simulink model "stdp_pattern3x3_training_2023noclock"  (R2024a)
settings: Solver=FixedStepAuto  StartTime=0.0  StopTime=2  FixedStep=0.000005  RelTol=1e-3
model workspace (MAT data in the model file):
  part1_v1 = 1
values from neighbouring files (symbols this model uses):
  full_pattern = load('Pattern4_250.CSV')    [model_setup4.m]
  max_weight2 = 255    [model_setup4.m]
  min_weight2 = 150    [model_setup4.m]
  Th_control_time2 = 0.02    [model_setup4.m]    (also in model_setup_test.m = 2)
  Th_minus_count2 = 10    [model_setup4.m]    (also in model_setup_test.m = 5)
  Th_plus_count2 = 20    [model_setup4.m]    (also in model_setup_test.m)
libraries: simulink x1
(part 9 of 9)

== matlab function stdp_pattern3x3_training_2023noclock/Post_Neuron1/MATLAB Function7 ==
  data: rc input; lateral_inhibition input; t input; inhibition_potential output
function inhibition_potential = fcn(rc, lateral_inhibition, t)

inhibition_potential = -lateral_inhibition * (exp(-(t)*rc));

== matlab function stdp_pattern3x3_training_2023noclock/Neuron1/MATLAB Function4 ==
  data: membrane_state input; t input; membrane_potential output
function membrane_potential = fcn(membrane_state, t)

membrane_potential = (membrane_state) * (exp(-(t)*0.015));

== matlab function stdp_pattern3x3_training_2023noclock/Neuron1/MATLAB Function5 ==
  data: t input; membrane_state input; membrane_potential output
function membrane_potential = fcn(t, membrane_state)

membrane_potential = (membrane_state) * 2.361128*(exp(-(t)*0.09)-0.6*exp(-(t+1)*0.04)) ;

== matlab function stdp_pattern3x3_training_2023noclock/Neuron1/Subsystem3/MATLAB Function ==
  data: u input; y output; min input; max input
function y = fcn(u, min, max)

if u<=min
    y=min;
elseif u>=max
    y=max;
else
    y=u;
end

== matlab function stdp_pattern3x3_training_2023noclock/Neuron5/MATLAB Function3 ==
  data: u input; y output
function y = fcn(u)

if u>=0
    y=1;
else
    y=0;
end

== matlab function stdp_pattern3x3_training_2023noclock/Neuron1/Subsystem3/MATLAB Function2 ==
  data: init_th input; y output; neuron_num input; before_threshold input
function y = fcn(init_th, neuron_num, before_threshold)

persistent n;

if isempty(n)
    n=init_th(neuron_num);
else
    n=before_threshold;
end

y=n;

== matlab function stdp_pattern3x3_training_2023noclock/Synapse1/rc_add2 ==
  data: tx input; initial_LTP input; pre_trace output; tau_LTP input
% rc_add2 (pre trace) - RC를 tau로 해석
function pre_trace = fcn(tx, initial_LTP, tau_LTP)
A   = initial_LTP(end);
tau = max(tau_LTP(end), eps);
pre_trace = A * exp(-tx / tau);

== matlab function stdp_pattern3x3_training_2023noclock/Subsystem1/MATLAB Function ==
  data: data input; y output; i input
function y = fcn(data, i)

j=1+i;
 y=data(j,:);
          

   
end

== matlab function stdp_pattern3x3_training_2023noclock/Neuron5/MATLAB Function4 ==
  data: membrane_state input; t input; membrane_potential output
function membrane_potential = fcn(membrane_state, t)

membrane_potential = (membrane_state) * (exp(-(t)*0.015));

== matlab function stdp_pattern3x3_training_2023noclock/Neuron5/MATLAB Function5 ==
  data: t input; membrane_state input; membrane_potential output
function membrane_potential = fcn(t, membrane_state)

membrane_potential = (membrane_state) * 2.361128*(exp(-(t)*0.09)-0.6*exp(-(t+1)*0.04)) ;

== matlab function stdp_pattern3x3_training_2023noclock/Neuron5/Subsystem3/MATLAB Function ==
  data: u input; y output; min input; max input
function y = fcn(u, min, max)

if u<=min
    y=min;
elseif u>=max
    y=max;
else
    y=u;
end

== matlab function stdp_pattern3x3_training_2023noclock/Neuron5/Subsystem3/MATLAB Function2 ==
  data: init_th input; y output; neuron_num input; before_threshold input
function y = fcn(init_th, neuron_num, before_threshold)

persistent n;

if isempty(n)
    n=init_th(neuron_num);
else
    n=before_threshold;
end

y=n;

== matlab function stdp_pattern3x3_training_2023noclock/Neuron6/MATLAB Function3 ==
  data: u input; y output
function y = fcn(u)

if u>=0
    y=1;
else
    y=0;
end

== matlab function stdp_pattern3x3_training_2023noclock/Neuron2/MATLAB Function3 ==
  data: u input; y output
function y = fcn(u)

if u>=0
    y=1;
else
    y=0;
end

== matlab function stdp_pattern3x3_training_2023noclock/Neuron6/MATLAB Function4 ==
  data: membrane_state input; t input; membrane_potential output
function membrane_potential = fcn(membrane_state, t)

membrane_potential = (membrane_state) * (exp(-(t)*0.015));

== matlab function stdp_pattern3x3_training_2023noclock/Neuron6/MATLAB Function5 ==
  data: t input; membrane_state input; membrane_potential output
function membrane_potential = fcn(t, membrane_state)

membrane_potential = (membrane_state) * 2.361128*(exp(-(t)*0.09)-0.6*exp(-(t+1)*0.04)) ;

== matlab function stdp_pattern3x3_training_2023noclock/Post_Neuron2/MATLAB Function3 ==
  data: membrane_state input; t input; membrane_potential output
function membrane_potential = fcn(membrane_state, t)

membrane_potential = (membrane_state) * (exp(-(t)*0.015));

== matlab function stdp_pattern3x3_training_2023noclock/Post_Neuron2/MATLAB Function4 ==
  data: t input; membrane_state input; membrane_potential output
function membrane_potential = fcn(t, membrane_state)

membrane_potential = (membrane_state) * 2.361128*(exp(-(t)*0.09)-0.6*exp(-(t+1)*0.04)) ;

== matlab function stdp_pattern3x3_training_2023noclock/Post_Neuron2/MATLAB Function7 ==
  data: rc input; lateral_inhibition input; t input; inhibition_potential output
function inhibition_potential = fcn(rc, lateral_inhibition, t)

inhibition_potential = -lateral_inhibition * (exp(-(t)*rc));

== matlab function stdp_pattern3x3_training_2023noclock/Post_Neuron2/Subsystem3/MATLAB Function ==
  data: u input; y output; min input; max input
function y = fcn(u, min, max)

if u<=min
    y=min;
elseif u>=max
    y=max;
else
    y=u;
end

== matlab function stdp_pattern3x3_training_2023noclock/Post_Neuron2/Subsystem3/MATLAB Function2 ==
  data: init_th input; y output; neuron_num input; before_threshold input
function y = fcn(init_th, neuron_num, before_threshold)

persistent n;

if isempty(n)
    n=init_th(neuron_num);
else
    n=before_threshold;
end

y=n;

== matlab function stdp_pattern3x3_training_2023noclock/Post_Neuron3/MATLAB Function1 ==
  data: u input; y output
function y = fcn(u)

if u>=0
    y=1;
else
    y=0;
end

== matlab function stdp_pattern3x3_training_2023noclock/Neuron2/MATLAB Function4 ==
  data: membrane_state input; t input; membrane_potential output
function membrane_potential = fcn(membrane_state, t)

membrane_potential = (membrane_state) * (exp(-(t)*0.015));

== matlab function stdp_pattern3x3_training_2023noclock/Post_Neuron3/MATLAB Function2 ==
  data: u input; y output
function y = fcn(u)
persistent k;
if isempty(k)
    k=0;
elseif u>0
    k=1;
end

y=k;

== matlab function stdp_pattern3x3_training_2023noclock/Post_Neuron3/MATLAB Function3 ==
  data: membrane_state input; t input; membrane_potential output
function membrane_potential = fcn(membrane_state, t)

membrane_potential = (membrane_state) * (exp(-(t)*0.015));

== matlab function stdp_pattern3x3_training_2023noclock/Post_Neuron3/MATLAB Function4 ==
  data: t input; membrane_state input; membrane_potential output
function membrane_potential = fcn(t, membrane_state)

membrane_potential = (membrane_state) * 2.361128*(exp(-(t)*0.09)-0.6*exp(-(t+1)*0.04)) ;

== matlab function stdp_pattern3x3_training_2023noclock/Post_Neuron3/MATLAB Function7 ==
  data: rc input; lateral_inhibition input; t input; inhibition_potential output
function inhibition_potential = fcn(rc, lateral_inhibition, t)

inhibition_potential = -lateral_inhibition * (exp(-(t)*rc));

== matlab function stdp_pattern3x3_training_2023noclock/Neuron6/Subsystem3/MATLAB Function ==
  data: u input; y output; min input; max input
function y = fcn(u, min, max)

if u<=min
    y=min;
elseif u>=max
    y=max;
else
    y=u;
end

== matlab function stdp_pattern3x3_training_2023noclock/Neuron6/Subsystem3/MATLAB Function2 ==
  data: init_th input; y output; neuron_num input; before_threshold input
function y = fcn(init_th, neuron_num, before_threshold)

persistent n;

if isempty(n)
    n=init_th(neuron_num);
else
    n=before_threshold;
end

y=n;

== matlab function stdp_pattern3x3_training_2023noclock/Synapse2/MATLAB Function1 ==
  data: init_weight input; y output; synapse_num input; before_weight input
function y = fcn(init_weight, synapse_num, before_weight)

persistent n;

if isempty(n)
    n=init_weight(synapse_num);
elseif before_weight>0
    n=before_weight;
end

y=n;

== matlab function stdp_pattern3x3_training_2023noclock/Synapse2/rc_add1 ==
  data: ty input; initial_LTD input; post_trace output; tau_LTD input
% rc_add1 (post trace) - RC를 tau로 해석
function post_trace = fcn(ty, initial_LTD, tau_LTD)
A   = initial_LTD(end);
tau = max(tau_LTD(end), eps);
post_trace = -A * exp(-ty / tau);

== matlab function stdp_pattern3x3_training_2023noclock/Synapse2/rc_add2 ==
  data: tx input; initial_LTP input; pre_trace output; tau_LTP input
% rc_add2 (pre trace) - RC를 tau로 해석
function pre_trace = fcn(tx, initial_LTP, tau_LTP)
A   = initial_LTP(end);
tau = max(tau_LTP(end), eps);
pre_trace = A * exp(-tx / tau);

== matlab function stdp_pattern3x3_training_2023noclock/Synapse3/MATLAB Function1 ==
  data: init_weight input; y output; synapse_num input; before_weight input
function y = fcn(init_weight, synapse_num, before_weight)

persistent n;

if isempty(n)
    n=init_weight(synapse_num);
elseif before_weight>0
    n=before_weight;
end

y=n;

== matlab function stdp_pattern3x3_training_2023noclock/Neuron2/MATLAB Function5 ==
  data: t input; membrane_state input; membrane_potential output
function membrane_potential = fcn(t, membrane_state)

membrane_potential = (membrane_state) * 2.361128*(exp(-(t)*0.09)-0.6*exp(-(t+1)*0.04)) ;

== matlab function stdp_pattern3x3_training_2023noclock/Synapse3/rc_add1 ==
  data: ty input; initial_LTD input; post_trace output; tau_LTD input
% rc_add1 (post trace) - RC를 tau로 해석
function post_trace = fcn(ty, initial_LTD, tau_LTD)
A   = initial_LTD(end);
tau = max(tau_LTD(end), eps);
post_trace = -A * exp(-ty / tau);

== matlab function stdp_pattern3x3_training_2023noclock/Synapse3/rc_add2 ==
  data: tx input; initial_LTP input; pre_trace output; tau_LTP input
% rc_add2 (pre trace) - RC를 tau로 해석
function pre_trace = fcn(tx, initial_LTP, tau_LTP)
A   = initial_LTP(end);
tau = max(tau_LTP(end), eps);
pre_trace = A * exp(-tx / tau);

== matlab function stdp_pattern3x3_training_2023noclock/Synapse4/MATLAB Function1 ==
  data: init_weight input; y output; synapse_num input; before_weight input
function y = fcn(init_weight, synapse_num, before_weight)

persistent n;

if isempty(n)
    n=init_weight(synapse_num);
elseif before_weight>0
    n=before_weight;
end

y=n;

== matlab function stdp_pattern3x3_training_2023noclock/Synapse4/rc_add1 ==
  data: ty input; initial_LTD input; post_trace output; tau_LTD input
% rc_add1 (post trace) - RC를 tau로 해석
function post_trace = fcn(ty, initial_LTD, tau_LTD)
A   = initial_LTD(end);
tau = max(tau_LTD(end), eps);
post_trace = -A * exp(-ty / tau);

== matlab function stdp_pattern3x3_training_2023noclock/Synapse4/rc_add2 ==
  data: tx input; initial_LTP input; pre_trace output; tau_LTP input
% rc_add2 (pre trace) - RC를 tau로 해석
function pre_trace = fcn(tx, initial_LTP, tau_LTP)
A   = initial_LTP(end);
tau = max(tau_LTP(end), eps);
pre_trace = A * exp(-tx / tau);

== matlab function stdp_pattern3x3_training_2023noclock/Synapse5/MATLAB Function1 ==
  data: init_weight input; y output; synapse_num input; before_weight input
function y = fcn(init_weight, synapse_num, before_weight)

persistent n;

if isempty(n)
    n=init_weight(synapse_num);
elseif before_weight>0
    n=before_weight;
end

y=n;

== matlab function stdp_pattern3x3_training_2023noclock/Synapse5/rc_add1 ==
  data: ty input; initial_LTD input; post_trace output; tau_LTD input
% rc_add1 (post trace) - RC를 tau로 해석
function post_trace = fcn(ty, initial_LTD, tau_LTD)
A   = initial_LTD(end);
tau = max(tau_LTD(end), eps);
post_trace = -A * exp(-ty / tau);

== matlab function stdp_pattern3x3_training_2023noclock/Synapse5/rc_add2 ==
  data: tx input; initial_LTP input; pre_trace output; tau_LTP input
% rc_add2 (pre trace) - RC를 tau로 해석
function pre_trace = fcn(tx, initial_LTP, tau_LTP)
A   = initial_LTP(end);
tau = max(tau_LTP(end), eps);
pre_trace = A * exp(-tx / tau);

== matlab function stdp_pattern3x3_training_2023noclock/Synapse6/MATLAB Function1 ==
  data: init_weight input; y output; synapse_num input; before_weight input
function y = fcn(init_weight, synapse_num, before_weight)

persistent n;

if isempty(n)
    n=init_weight(synapse_num);
elseif before_weight>0
    n=before_weight;
end

y=n;

== matlab function stdp_pattern3x3_training_2023noclock/Post_Neuron2/MATLAB Function1 ==
  data: u input; y output
function y = fcn(u)

if u>=0
    y=1;
else
    y=0;
end

== matlab function stdp_pattern3x3_training_2023noclock/Synapse6/rc_add1 ==
  data: ty input; initial_LTD input; post_trace output; tau_LTD input
% rc_add1 (post trace) - RC를 tau로 해석
function post_trace = fcn(ty, initial_LTD, tau_LTD)
A   = initial_LTD(end);
tau = max(tau_LTD(end), eps);
post_trace = -A * exp(-ty / tau);

== matlab function stdp_pattern3x3_training_2023noclock/Synapse6/rc_add2 ==
  data: tx input; initial_LTP input; pre_trace output; tau_LTP input
% rc_add2 (pre trace) - RC를 tau로 해석
function pre_trace = fcn(tx, initial_LTP, tau_LTP)
A   = initial_LTP(end);
tau = max(tau_LTP(end), eps);
pre_trace = A * exp(-tx / tau);

== matlab function stdp_pattern3x3_training_2023noclock/Synapse7/MATLAB Function1 ==
  data: init_weight input; y output; synapse_num input; before_weight input
function y = fcn(init_weight, synapse_num, before_weight)

persistent n;

if isempty(n)
    n=init_weight(synapse_num);
elseif before_weight>0
    n=before_weight;
end

y=n;

== matlab function stdp_pattern3x3_training_2023noclock/Synapse7/rc_add1 ==
  data: ty input; initial_LTD input; post_trace output; tau_LTD input
% rc_add1 (post trace) - RC를 tau로 해석
function post_trace = fcn(ty, initial_LTD, tau_LTD)
A   = initial_LTD(end);
tau = max(tau_LTD(end), eps);
post_trace = -A * exp(-ty / tau);

== matlab function stdp_pattern3x3_training_2023noclock/Synapse7/rc_add2 ==
  data: tx input; initial_LTP input; pre_trace output; tau_LTP input
% rc_add2 (pre trace) - RC를 tau로 해석
function pre_trace = fcn(tx, initial_LTP, tau_LTP)
A   = initial_LTP(end);
tau = max(tau_LTP(end), eps);
pre_trace = A * exp(-tx / tau);

== matlab function stdp_pattern3x3_training_2023noclock/Synapse8/MATLAB Function1 ==
  data: init_weight input; y output; synapse_num input; before_weight input
function y = fcn(init_weight, synapse_num, before_weight)

persistent n;

if isempty(n)
    n=init_weight(synapse_num);
elseif before_weight>0
    n=before_weight;
end

y=n;

== matlab function stdp_pattern3x3_training_2023noclock/Synapse8/rc_add1 ==
  data: ty input; initial_LTD input; post_trace output; tau_LTD input
% rc_add1 (post trace) - RC를 tau로 해석
function post_trace = fcn(ty, initial_LTD, tau_LTD)
A   = initial_LTD(end);
tau = max(tau_LTD(end), eps);
post_trace = -A * exp(-ty / tau);

== matlab function stdp_pattern3x3_training_2023noclock/Post_Neuron2/MATLAB Function2 ==
  data: u input; y output
function y = fcn(u)
persistent k;
if isempty(k)
    k=0;
elseif u>0
    k=1;
end

y=k;

== matlab function stdp_pattern3x3_training_2023noclock/Synapse8/rc_add2 ==
  data: tx input; initial_LTP input; pre_trace output; tau_LTP input
% rc_add2 (pre trace) - RC를 tau로 해석
function pre_trace = fcn(tx, initial_LTP, tau_LTP)
A   = initial_LTP(end);
tau = max(tau_LTP(end), eps);
pre_trace = A * exp(-tx / tau);

== matlab function stdp_pattern3x3_training_2023noclock/Synapse9/MATLAB Function1 ==
  data: init_weight input; y output; synapse_num input; before_weight input
function y = fcn(init_weight, synapse_num, before_weight)

persistent n;

if isempty(n)
    n=init_weight(synapse_num);
elseif before_weight>0
    n=before_weight;
end

y=n;

== matlab function stdp_pattern3x3_training_2023noclock/Synapse9/rc_add1 ==
  data: ty input; initial_LTD input; post_trace output; tau_LTD input
% rc_add1 (post trace) - RC를 tau로 해석
function post_trace = fcn(ty, initial_LTD, tau_LTD)
A   = initial_LTD(end);
tau = max(tau_LTD(end), eps);
post_trace = -A * exp(-ty / tau);

== matlab function stdp_pattern3x3_training_2023noclock/Synapse9/rc_add2 ==
  data: tx input; initial_LTP input; pre_trace output; tau_LTP input
% rc_add2 (pre trace) - RC를 tau로 해석
function pre_trace = fcn(tx, initial_LTP, tau_LTP)
A   = initial_LTP(end);
tau = max(tau_LTP(end), eps);
pre_trace = A * exp(-tx / tau);

== matlab function stdp_pattern3x3_training_2023noclock/Synapse10/MATLAB Function1 ==
  data: init_weight input; y output; synapse_num input; before_weight input
function y = fcn(init_weight, synapse_num, before_weight)

persistent n;

if isempty(n)
    n=init_weight(synapse_num);
elseif before_weight>0
    n=before_weight;
end

y=n;

== matlab function stdp_pattern3x3_training_2023noclock/Synapse10/rc_add1 ==
  data: ty input; initial_LTD input; post_trace output; tau_LTD input
% rc_add1 (post trace) - RC를 tau로 해석
function post_trace = fcn(ty, initial_LTD, tau_LTD)
A   = initial_LTD(end);
tau = max(tau_LTD(end), eps);
post_trace = -A * exp(-ty / tau);

== matlab function stdp_pattern3x3_training_2023noclock/Synapse10/rc_add2 ==
  data: tx input; initial_LTP input; pre_trace output; tau_LTP input
% rc_add2 (pre trace) - RC를 tau로 해석
function pre_trace = fcn(tx, initial_LTP, tau_LTP)
A   = initial_LTP(end);
tau = max(tau_LTP(end), eps);
pre_trace = A * exp(-tx / tau);

== matlab function stdp_pattern3x3_training_2023noclock/Synapse11/MATLAB Function1 ==
  data: init_weight input; y output; synapse_num input; before_weight input
function y = fcn(init_weight, synapse_num, before_weight)

persistent n;

if isempty(n)
    n=init_weight(synapse_num);
elseif before_weight>0
    n=before_weight;
end

y=n;

== matlab function stdp_pattern3x3_training_2023noclock/Neuron2/Subsystem3/MATLAB Function ==
  data: u input; y output; min input; max input
function y = fcn(u, min, max)

if u<=min
    y=min;
elseif u>=max
    y=max;
else
    y=u;
end

== matlab function stdp_pattern3x3_training_2023noclock/Synapse11/rc_add1 ==
  data: ty input; initial_LTD input; post_trace output; tau_LTD input
% rc_add1 (post trace) - RC를 tau로 해석
function post_trace = fcn(ty, initial_LTD, tau_LTD)
A   = initial_LTD(end);
tau = max(tau_LTD(end), eps);
post_trace = -A * exp(-ty / tau);

== matlab function stdp_pattern3x3_training_2023noclock/Synapse11/rc_add2 ==
  data: tx input; initial_LTP input; pre_trace output; tau_LTP input
% rc_add2 (pre trace) - RC를 tau로 해석
function pre_trace = fcn(tx, initial_LTP, tau_LTP)
A   = initial_LTP(end);
tau = max(tau_LTP(end), eps);
pre_trace = A * exp(-tx / tau);

== matlab function stdp_pattern3x3_training_2023noclock/Synapse12/MATLAB Function1 ==
  data: init_weight input; y output; synapse_num input; before_weight input
function y = fcn(init_weight, synapse_num, before_weight)

persistent n;

if isempty(n)
    n=init_weight(synapse_num);
elseif before_weight>0
    n=before_weight;
end

y=n;

== matlab function stdp_pattern3x3_training_2023noclock/Synapse12/rc_add1 ==
  data: ty input; initial_LTD input; post_trace output; tau_LTD input
% rc_add1 (post trace) - RC를 tau로 해석
function post_trace = fcn(ty, initial_LTD, tau_LTD)
A   = initial_LTD(end);
tau = max(tau_LTD(end), eps);
post_trace = -A * exp(-ty / tau);

== matlab function stdp_pattern3x3_training_2023noclock/Synapse1/MATLAB Function1 ==
  data: init_weight input; y output; synapse_num input; before_weight input
function y = fcn(init_weight, synapse_num, before_weight)

persistent n;

if isempty(n)
    n=init_weight(synapse_num);
elseif before_weight>0
    n=before_weight;
end

y=n;

== matlab function stdp_pattern3x3_training_2023noclock/Synapse12/rc_add2 ==
  data: tx input; initial_LTP input; pre_trace output; tau_LTP input
% rc_add2 (pre trace) - RC를 tau로 해석
function pre_trace = fcn(tx, initial_LTP, tau_LTP)
A   = initial_LTP(end);
tau = max(tau_LTP(end), eps);
pre_trace = A * exp(-tx / tau);

== matlab function stdp_pattern3x3_training_2023noclock/Synapse13/MATLAB Function1 ==
  data: init_weight input; y output; synapse_num input; before_weight input
function y = fcn(init_weight, synapse_num, before_weight)

persistent n;

if isempty(n)
    n=init_weight(synapse_num);
elseif before_weight>0
    n=before_weight;
end

y=n;

== matlab function stdp_pattern3x3_training_2023noclock/Synapse13/rc_add1 ==
  data: ty input; initial_LTD input; post_trace output; tau_LTD input
% rc_add1 (post trace) - RC를 tau로 해석
function post_trace = fcn(ty, initial_LTD, tau_LTD)
A   = initial_LTD(end);
tau = max(tau_LTD(end), eps);
post_trace = -A * exp(-ty / tau);

== matlab function stdp_pattern3x3_training_2023noclock/Synapse13/rc_add2 ==
  data: tx input; initial_LTP input; pre_trace output; tau_LTP input
% rc_add2 (pre trace) - RC를 tau로 해석
function pre_trace = fcn(tx, initial_LTP, tau_LTP)
A   = initial_LTP(end);
tau = max(tau_LTP(end), eps);
pre_trace = A * exp(-tx / tau);

== matlab function stdp_pattern3x3_training_2023noclock/Synapse14/MATLAB Function1 ==
  data: init_weight input; y output; synapse_num input; before_weight input
function y = fcn(init_weight, synapse_num, before_weight)

persistent n;

if isempty(n)
    n=init_weight(synapse_num);
elseif before_weight>0
    n=before_weight;
end

y=n;

== matlab function stdp_pattern3x3_training_2023noclock/Neuron2/Subsystem3/MATLAB Function2 ==
  data: init_th input; y output; neuron_num input; before_threshold input
function y = fcn(init_th, neuron_num, before_threshold)

persistent n;

if isempty(n)
    n=init_th(neuron_num);
else
    n=before_threshold;
end

y=n;

== matlab function stdp_pattern3x3_training_2023noclock/Synapse14/rc_add1 ==
  data: ty input; initial_LTD input; post_trace output; tau_LTD input
% rc_add1 (post trace) - RC를 tau로 해석
function post_trace = fcn(ty, initial_LTD, tau_LTD)
A   = initial_LTD(end);
tau = max(tau_LTD(end), eps);
post_trace = -A * exp(-ty / tau);

== matlab function stdp_pattern3x3_training_2023noclock/Synapse14/rc_add2 ==
  data: tx input; initial_LTP input; pre_trace output; tau_LTP input
% rc_add2 (pre trace) - RC를 tau로 해석
function pre_trace = fcn(tx, initial_LTP, tau_LTP)
A   = initial_LTP(end);
tau = max(tau_LTP(end), eps);
pre_trace = A * exp(-tx / tau);

== matlab function stdp_pattern3x3_training_2023noclock/Synapse15/MATLAB Function1 ==
  data: init_weight input; y output; synapse_num input; before_weight input
function y = fcn(init_weight, synapse_num, before_weight)

persistent n;

if isempty(n)
    n=init_weight(synapse_num);
elseif before_weight>0
    n=before_weight;
end

y=n;

== matlab function stdp_pattern3x3_training_2023noclock/Synapse15/rc_add1 ==
  data: ty input; initial_LTD input; post_trace output; tau_LTD input
% rc_add1 (post trace) - RC를 tau로 해석
function post_trace = fcn(ty, initial_LTD, tau_LTD)
A   = initial_LTD(end);
tau = max(tau_LTD(end), eps);
post_trace = -A * exp(-ty / tau);

== matlab function stdp_pattern3x3_training_2023noclock/Synapse15/rc_add2 ==
  data: tx input; initial_LTP input; pre_trace output; tau_LTP input
% rc_add2 (pre trace) - RC를 tau로 해석
function pre_trace = fcn(tx, initial_LTP, tau_LTP)
A   = initial_LTP(end);
tau = max(tau_LTP(end), eps);
pre_trace = A * exp(-tx / tau);

== matlab function stdp_pattern3x3_training_2023noclock/Synapse16/MATLAB Function1 ==
  data: init_weight input; y output; synapse_num input; before_weight input
function y = fcn(init_weight, synapse_num, before_weight)

persistent n;

if isempty(n)
    n=init_weight(synapse_num);
elseif before_weight>0
    n=before_weight;
end

y=n;

== matlab function stdp_pattern3x3_training_2023noclock/Synapse16/rc_add1 ==
  data: ty input; initial_LTD input; post_trace output; tau_LTD input
% rc_add1 (post trace) - RC를 tau로 해석
function post_trace = fcn(ty, initial_LTD, tau_LTD)
A   = initial_LTD(end);
tau = max(tau_LTD(end), eps);
post_trace = -A * exp(-ty / tau);

== matlab function stdp_pattern3x3_training_2023noclock/Synapse16/rc_add2 ==
  data: tx input; initial_LTP input; pre_trace output; tau_LTP input
% rc_add2 (pre trace) - RC를 tau로 해석
function pre_trace = fcn(tx, initial_LTP, tau_LTP)
A   = initial_LTP(end);
tau = max(tau_LTP(end), eps);
pre_trace = A * exp(-tx / tau);

== matlab function stdp_pattern3x3_training_2023noclock/Synapse17/MATLAB Function1 ==
  data: init_weight input; y output; synapse_num input; before_weight input
function y = fcn(init_weight, synapse_num, before_weight)

persistent n;

if isempty(n)
    n=init_weight(synapse_num);
elseif before_weight>0
    n=before_weight;
end

y=n;

== matlab function stdp_pattern3x3_training_2023noclock/Synapse17/rc_add1 ==
  data: ty input; initial_LTD input; post_trace output; tau_LTD input
% rc_add1 (post trace) - RC를 tau로 해석
function post_trace = fcn(ty, initial_LTD, tau_LTD)
A   = initial_LTD(end);
tau = max(tau_LTD(end), eps);
post_trace = -A * exp(-ty / tau);

== matlab function stdp_pattern3x3_training_2023noclock/Neuron3/MATLAB Function3 ==
  data: u input; y output
function y = fcn(u)

if u>=0
    y=1;
else
    y=0;
end

== matlab function stdp_pattern3x3_training_2023noclock/Synapse17/rc_add2 ==
  data: tx input; initial_LTP input; pre_trace output; tau_LTP input
% rc_add2 (pre trace) - RC를 tau로 해석
function pre_trace = fcn(tx, initial_LTP, tau_LTP)
A   = initial_LTP(end);
tau = max(tau_LTP(end), eps);
pre_trace = A * exp(-tx / tau);

== matlab function stdp_pattern3x3_training_2023noclock/Synapse18/MATLAB Function1 ==
  data: init_weight input; y output; synapse_num input; before_weight input
function y = fcn(init_weight, synapse_num, before_weight)

persistent n;

if isempty(n)
    n=init_weight(synapse_num);
elseif before_weight>0
    n=before_weight;
end

y=n;

== matlab function stdp_pattern3x3_training_2023noclock/Synapse18/rc_add1 ==
  data: ty input; initial_LTD input; post_trace output; tau_LTD input
% rc_add1 (post trace) - RC를 tau로 해석
function post_trace = fcn(ty, initial_LTD, tau_LTD)
A   = initial_LTD(end);
tau = max(tau_LTD(end), eps);
post_trace = -A * exp(-ty / tau);

== matlab function stdp_pattern3x3_training_2023noclock/Synapse18/rc_add2 ==
  data: tx input; initial_LTP input; pre_trace output; tau_LTP input
% rc_add2 (pre trace) - RC를 tau로 해석
function pre_trace = fcn(tx, initial_LTP, tau_LTP)
A   = initial_LTP(end);
tau = max(tau_LTP(end), eps);
pre_trace = A * exp(-tx / tau);

== matlab function stdp_pattern3x3_training_2023noclock/Synapse19/MATLAB Function1 ==
  data: init_weight input; y output; synapse_num input; before_weight input
function y = fcn(init_weight, synapse_num, before_weight)

persistent n;

if isempty(n)
    n=init_weight(synapse_num);
elseif before_weight>0
    n=before_weight;
end

y=n;

== matlab function stdp_pattern3x3_training_2023noclock/Synapse19/rc_add1 ==
  data: ty input; initial_LTD input; post_trace output; tau_LTD input
% rc_add1 (post trace) - RC를 tau로 해석
function post_trace = fcn(ty, initial_LTD, tau_LTD)
A   = initial_LTD(end);
tau = max(tau_LTD(end), eps);
post_trace = -A * exp(-ty / tau);

== matlab function stdp_pattern3x3_training_2023noclock/Synapse19/rc_add2 ==
  data: tx input; initial_LTP input; pre_trace output; tau_LTP input
% rc_add2 (pre trace) - RC를 tau로 해석
function pre_trace = fcn(tx, initial_LTP, tau_LTP)
A   = initial_LTP(end);
tau = max(tau_LTP(end), eps);
pre_trace = A * exp(-tx / tau);

== matlab function stdp_pattern3x3_training_2023noclock/Synapse20/MATLAB Function1 ==
  data: init_weight input; y output; synapse_num input; before_weight input
function y = fcn(init_weight, synapse_num, before_weight)

persistent n;

if isempty(n)
    n=init_weight(synapse_num);
elseif before_weight>0
    n=before_weight;
end

y=n;

== matlab function stdp_pattern3x3_training_2023noclock/Neuron3/MATLAB Function4 ==
  data: membrane_state input; t input; membrane_potential output
function membrane_potential = fcn(membrane_state, t)

membrane_potential = (membrane_state) * (exp(-(t)*0.015));

== matlab function stdp_pattern3x3_training_2023noclock/Synapse20/rc_add1 ==
  data: ty input; initial_LTD input; post_trace output; tau_LTD input
% rc_add1 (post trace) - RC를 tau로 해석
function post_trace = fcn(ty, initial_LTD, tau_LTD)
A   = initial_LTD(end);
tau = max(tau_LTD(end), eps);
post_trace = -A * exp(-ty / tau);

== matlab function stdp_pattern3x3_training_2023noclock/Synapse20/rc_add2 ==
  data: tx input; initial_LTP input; pre_trace output; tau_LTP input
% rc_add2 (pre trace) - RC를 tau로 해석
function pre_trace = fcn(tx, initial_LTP, tau_LTP)
A   = initial_LTP(end);
tau = max(tau_LTP(end), eps);
pre_trace = A * exp(-tx / tau);

== matlab function stdp_pattern3x3_training_2023noclock/Synapse21/MATLAB Function1 ==
  data: init_weight input; y output; synapse_num input; before_weight input
function y = fcn(init_weight, synapse_num, before_weight)

persistent n;

if isempty(n)
    n=init_weight(synapse_num);
elseif before_weight>0
    n=before_weight;
end

y=n;

== matlab function stdp_pattern3x3_training_2023noclock/Synapse21/rc_add1 ==
  data: ty input; initial_LTD input; post_trace output; tau_LTD input
% rc_add1 (post trace) - RC를 tau로 해석
function post_trace = fcn(ty, initial_LTD, tau_LTD)
A   = initial_LTD(end);
tau = max(tau_LTD(end), eps);
post_trace = -A * exp(-ty / tau);

== matlab function stdp_pattern3x3_training_2023noclock/Synapse21/rc_add2 ==
  data: tx input; initial_LTP input; pre_trace output; tau_LTP input
% rc_add2 (pre trace) - RC를 tau로 해석
function pre_trace = fcn(tx, initial_LTP, tau_LTP)
A   = initial_LTP(end);
tau = max(tau_LTP(end), eps);
pre_trace = A * exp(-tx / tau);

== matlab function stdp_pattern3x3_training_2023noclock/Synapse22/MATLAB Function1 ==
  data: init_weight input; y output; synapse_num input; before_weight input
function y = fcn(init_weight, synapse_num, before_weight)

persistent n;

if isempty(n)
    n=init_weight(synapse_num);
elseif before_weight>0
    n=before_weight;
end

y=n;

== matlab function stdp_pattern3x3_training_2023noclock/Synapse22/rc_add1 ==
  data: ty input; initial_LTD input; post_trace output; tau_LTD input
% rc_add1 (post trace) - RC를 tau로 해석
function post_trace = fcn(ty, initial_LTD, tau_LTD)
A   = initial_LTD(end);
tau = max(tau_LTD(end), eps);
post_trace = -A * exp(-ty / tau);

== matlab function stdp_pattern3x3_training_2023noclock/Synapse22/rc_add2 ==
  data: tx input; initial_LTP input; pre_trace output; tau_LTP input
% rc_add2 (pre trace) - RC를 tau로 해석
function pre_trace = fcn(tx, initial_LTP, tau_LTP)
A   = initial_LTP(end);
tau = max(tau_LTP(end), eps);
pre_trace = A * exp(-tx / tau);

== matlab function stdp_pattern3x3_training_2023noclock/Synapse23/MATLAB Function1 ==
  data: init_weight input; y output; synapse_num input; before_weight input
function y = fcn(init_weight, synapse_num, before_weight)

persistent n;

if isempty(n)
    n=init_weight(synapse_num);
elseif before_weight>0
    n=before_weight;
end

y=n;

== matlab function stdp_pattern3x3_training_2023noclock/Neuron3/MATLAB Function5 ==
  data: t input; membrane_state input; membrane_potential output
function membrane_potential = fcn(t, membrane_state)

membrane_potential = (membrane_state) * 2.361128*(exp(-(t)*0.09)-0.6*exp(-(t+1)*0.04)) ;

== matlab function stdp_pattern3x3_training_2023noclock/Synapse23/rc_add1 ==
  data: ty input; initial_LTD input; post_trace output; tau_LTD input
% rc_add1 (post trace) - RC를 tau로 해석
function post_trace = fcn(ty, initial_LTD, tau_LTD)
A   = initial_LTD(end);
tau = max(tau_LTD(end), eps);
post_trace = -A * exp(-ty / tau);

== matlab function stdp_pattern3x3_training_2023noclock/Synapse23/rc_add2 ==
  data: tx input; initial_LTP input; pre_trace output; tau_LTP input
% rc_add2 (pre trace) - RC를 tau로 해석
function pre_trace = fcn(tx, initial_LTP, tau_LTP)
A   = initial_LTP(end);
tau = max(tau_LTP(end), eps);
pre_trace = A * exp(-tx / tau);

== matlab function stdp_pattern3x3_training_2023noclock/Synapse24/MATLAB Function1 ==
  data: init_weight input; y output; synapse_num input; before_weight input
function y = fcn(init_weight, synapse_num, before_weight)

persistent n;

if isempty(n)
    n=init_weight(synapse_num);
elseif before_weight>0
    n=before_weight;
end

y=n;

== matlab function stdp_pattern3x3_training_2023noclock/Synapse24/rc_add1 ==
  data: ty input; initial_LTD input; post_trace output; tau_LTD input
% rc_add1 (post trace) - RC를 tau로 해석
function post_trace = fcn(ty, initial_LTD, tau_LTD)
A   = initial_LTD(end);
tau = max(tau_LTD(end), eps);
post_trace = -A * exp(-ty / tau);

== matlab function stdp_pattern3x3_training_2023noclock/Synapse24/rc_add2 ==
  data: tx input; initial_LTP input; pre_trace output; tau_LTP input
% rc_add2 (pre trace) - RC를 tau로 해석
function pre_trace = fcn(tx, initial_LTP, tau_LTP)
A   = initial_LTP(end);
tau = max(tau_LTP(end), eps);
pre_trace = A * exp(-tx / tau);

== matlab function stdp_pattern3x3_training_2023noclock/Synapse25/MATLAB Function1 ==
  data: init_weight input; y output; synapse_num input; before_weight input
function y = fcn(init_weight, synapse_num, before_weight)

persistent n;

if isempty(n)
    n=init_weight(synapse_num);
elseif before_weight>0
    n=before_weight;
end

y=n;

== matlab function stdp_pattern3x3_training_2023noclock/Synapse25/rc_add1 ==
  data: ty input; initial_LTD input; post_trace output; tau_LTD input
% rc_add1 (post trace) - RC를 tau로 해석
function post_trace = fcn(ty, initial_LTD, tau_LTD)
A   = initial_LTD(end);
tau = max(tau_LTD(end), eps);
post_trace = -A * exp(-ty / tau);

== matlab function stdp_pattern3x3_training_2023noclock/Synapse25/rc_add2 ==
  data: tx input; initial_LTP input; pre_trace output; tau_LTP input
% rc_add2 (pre trace) - RC를 tau로 해석
function pre_trace = fcn(tx, initial_LTP, tau_LTP)
A   = initial_LTP(end);
tau = max(tau_LTP(end), eps);
pre_trace = A * exp(-tx / tau);

== matlab function stdp_pattern3x3_training_2023noclock/Synapse26/MATLAB Function1 ==
  data: init_weight input; y output; synapse_num input; before_weight input
function y = fcn(init_weight, synapse_num, before_weight)

persistent n;

if isempty(n)
    n=init_weight(synapse_num);
elseif before_weight>0
    n=before_weight;
end

y=n;

== matlab function stdp_pattern3x3_training_2023noclock/Neuron3/Subsystem3/MATLAB Function ==
  data: u input; y output; min input; max input
function y = fcn(u, min, max)

if u<=min
    y=min;
elseif u>=max
    y=max;
else
    y=u;
end

== matlab function stdp_pattern3x3_training_2023noclock/Synapse26/rc_add1 ==
  data: ty input; initial_LTD input; post_trace output; tau_LTD input
% rc_add1 (post trace) - RC를 tau로 해석
function post_trace = fcn(ty, initial_LTD, tau_LTD)
A   = initial_LTD(end);
tau = max(tau_LTD(end), eps);
post_trace = -A * exp(-ty / tau);

== matlab function stdp_pattern3x3_training_2023noclock/Synapse26/rc_add2 ==
  data: tx input; initial_LTP input; pre_trace output; tau_LTP input
% rc_add2 (pre trace) - RC를 tau로 해석
function pre_trace = fcn(tx, initial_LTP, tau_LTP)
A   = initial_LTP(end);
tau = max(tau_LTP(end), eps);
pre_trace = A * exp(-tx / tau);
